simulink model "PID_Gains"  (Simulink 6.6)
settings: Solver=ode45  StartTime=0.0  StopTime=200  RelTol=1e-3
InitFcn:
  | L=0.15;
  | Kwf=0.00011712;
  | Izz = 0.02;
  | alpha = -2;
  | Kvwdot=3242;
libraries: simulink_extras x1
settings Model: Creator=Cooch  LastModifiedBy=Cooch

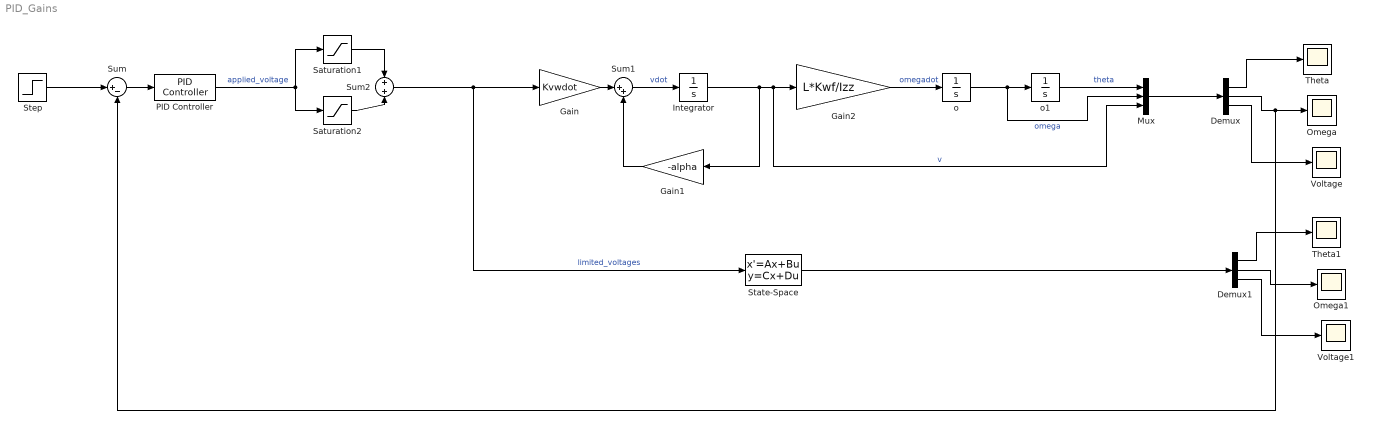
== system PID_Gains ==
  Demux : Demux  Outputs=3
  Demux1 : Demux  Outputs=3
  Gain : Gain  Gain=Kvwdot
  Gain1 : Gain  Orientation=left  Gain=-alpha
  Gain2 : Gain  Gain=L*Kwf/Izz
  Integrator : Integrator
  Mux : Mux  Inputs=3
  Omega : Scope
      settings: TimeRange=200  YMin=0  YMax=0.5
  Omega1 : Scope
      settings: TimeRange=200  YMin=0  YMax=0.5
  PID Controller : simulink_extras/Additional Linear/PID Controller  SystemSampleTime=-1  P=1  I=1  D=1
  Saturation1 : Saturate  UpperLimit=14  LowerLimit=10
  Saturation2 : Saturate  UpperLimit=-10  LowerLimit=-14
  State-Space : StateSpace  A=[0 1 0; 0 0 L*Kwf/Izz; 0 0 -alpha]  B=[0; 0; Kvwdot]  C=eye(3)  D=[0;0;0]  X0=[0;0;0]
  Step : Step  Time=0  After=20*2*pi()/60  SampleTime=0
  Sum : Sum  Inputs=|+-
  Sum1 : Sum  Inputs=|++
  Sum2 : Sum  Inputs=+|+
  Theta : Scope
      settings: TimeRange=200  YMin=0  YMax=0.5  SaveName=ScopeData2
  Theta1 : Scope
      settings: TimeRange=200  YMin=0  YMax=0.5  SaveName=ScopeData4
  Voltage : Scope
      settings: TimeRange=200  YMin=0  YMax=0.5  SaveName=ScopeData3
  Voltage1 : Scope
      settings: TimeRange=200  YMin=0  YMax=0.5  SaveName=ScopeData5
  o : Integrator
  o1 : Integrator
  wires:
  Step/1 -> Sum/1
  Sum/1 -> PID Controller/1
  Sum2/1 -> Gain/1, State-Space/1  "limited_voltages"
  PID Controller/1 -> Saturation1/1, Saturation2/1  "applied_voltage"
  Gain/1 -> Sum1/1
  Sum1/1 -> Integrator/1  "vdot"
  Gain1/1 -> Sum1/2
  Gain2/1 -> o/1  "omegadot"
  o/1 -> o1/1, Mux/2  "omega"
  o1/1 -> Mux/1  "theta"
  Demux/1 -> Theta/1
  Demux/2 -> Omega/1, Sum/2
  Demux/3 -> Voltage/1
  Mux/1 -> Demux/1
  Demux1/1 -> Theta1/1
  Demux1/2 -> Omega1/1
  Demux1/3 -> Voltage1/1
  State-Space/1 -> Demux1/1
  Integrator/1 -> Gain1/1, Gain2/1, Mux/3  "v"
  Saturation1/1 -> Sum2/1
  Saturation2/1 -> Sum2/2
